simulink model "DB_2"  (R2018a)
settings: Solver=VariableStepAuto  StartTime=0.0  StopTime=10.0  RelTol=1e-3
settings Model: Creator=valen  LastModifiedBy=valen

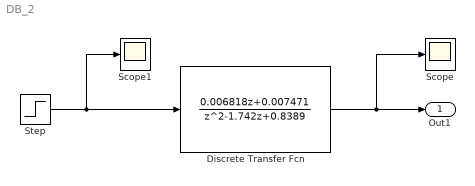
== system DB_2 ==
  Discrete Transfer Fcn : DiscreteTransferFcn  Numerator=[0.006818 0.007471]  Denominator=[1 -1.742 0.8389]
  Scope : Scope
  Scope1 : Scope
  Step : Step  Time=0.1  After=440  SampleTime=0
  Out1 : Outport
  wires:
  Discrete Transfer Fcn/1 -> Scope/1, Out1/1
  Step/1 -> Scope1/1, Discrete Transfer Fcn/1
